simulink model "FLController_a_diff"  (R2018a)
settings: Solver=FixedStepAuto  StartTime=0.0  StopTime=10  MaxStep=0.01  RelTol=1e-4  EnableMultiTasking=on
libraries: fuzblock x4
settings Model: Creator=G  LastModifiedBy=G
settings DataIOCC: LimitDataPoints=on  SaveOutput=off  SaveTime=off
settings OptimizationCC: ExpressionDepthLimit=2147483647  LifeSpan=1
settings DebuggingCC: UnderspecifiedInitializationDetection=Classic  MergeDetectMultiDrivingBlocksExec=none  FcnCallInpInsideContextMsg=warning  AllowSymbolicDim=off  StateNameClashWarn=warning  SFUnexpectedBacktrackingDiag=warning  SFNoUnconditionalDefaultTransitionDiag=warning  SFExecutionAtInitializationDiag=none
settings CodeAppCC: StateflowObjectComments=on
settings GRTTargetCC: TargetLangStandard=C89/C90 (ANSI)  GeneratePreprocessorConditionals=Disable all  CombineOutputUpdateFcns=off  GRTInterface=on

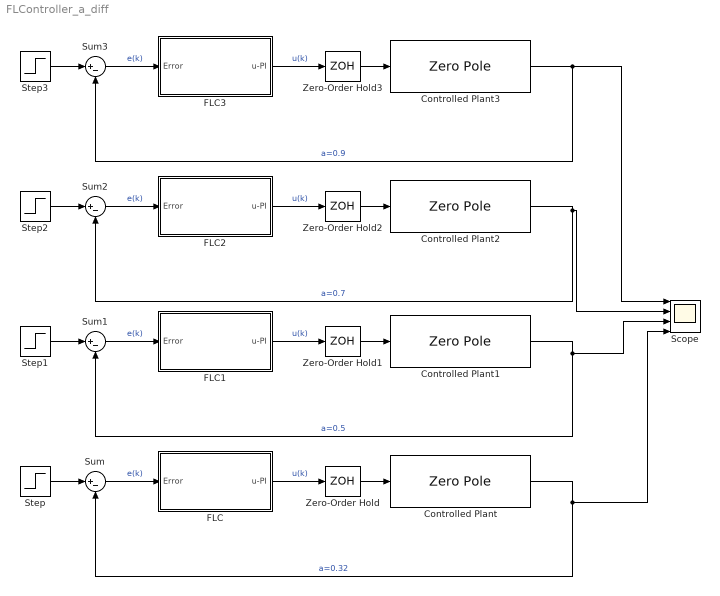
== system FLController_a_diff ==
  Controlled Plant{,1..3} (4 alike) : ZeroPole  Zeros=[]  Poles=[-0.1 -10]  Gain=25
  FLC : Subsystem
  FLC1 : Subsystem
  FLC2 : Subsystem
  FLC3 : Subsystem
  Scope : Scope  NumInputPorts=4
  Step{,1..3} (4 alike) : Step  Time=0  After=50  SampleTime=0.01
  Sum{,1..3} (4 alike) : Sum  Inputs=|+-
  Zero-Order Hold{,1..3} (4 alike) : ZeroOrderHold  SampleTime=-1
  wires:
  Controlled Plant/1 -> Scope/4, Sum/2  "a=0.32"
  Sum/1 -> FLC/1(Error)  "e(k)"
  FLC/1(u-PI) -> Zero-Order Hold/1  "u(k)"
  Zero-Order Hold/1 -> Controlled Plant/1
  Step/1 -> Sum/1
  Step1/1 -> Sum1/1
  Zero-Order Hold1/1 -> Controlled Plant1/1
  FLC1/1(u-PI) -> Zero-Order Hold1/1  "u(k)"
  Sum1/1 -> FLC1/1(Error)  "e(k)"
  Controlled Plant1/1 -> Scope/3, Sum1/2  "a=0.5"
  Step2/1 -> Sum2/1
  Zero-Order Hold2/1 -> Controlled Plant2/1
  FLC2/1(u-PI) -> Zero-Order Hold2/1  "u(k)"
  Sum2/1 -> FLC2/1(Error)  "e(k)"
  Controlled Plant2/1 -> Scope/2, Sum2/2  "a=0.7"
  Step3/1 -> Sum3/1
  Zero-Order Hold3/1 -> Controlled Plant3/1
  FLC3/1(u-PI) -> Zero-Order Hold3/1  "u(k)"
  Sum3/1 -> FLC3/1(Error)  "e(k)"
  Controlled Plant3/1 -> Scope/1, Sum3/2  "a=0.9"

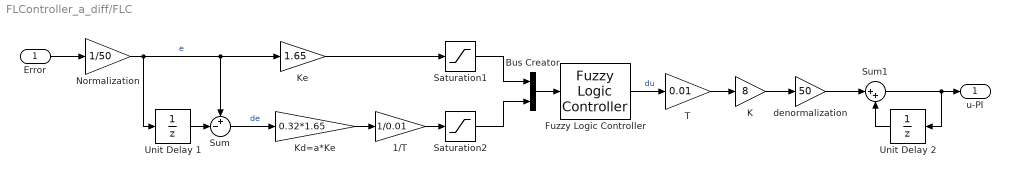
== system FLController_a_diff/FLC ==
  Error : Inport
  "1/T " : Gain  Gain=1/0.01
  Bus Creator : BusCreator  Inputs=2
  Fuzzy Logic Controller : fuzblock/Fuzzy Logic  Controller  FIS='FLController.fis'  OutputSampleNumber=101  DataType=double  FuzzifiedInputs=off  RuleFiringStrengths=off  RuleOutputs=off  AggregatedOutputs=off  SimulateUsing=Interpreted execution  OutOfRangeInputValueMessage=warning  NoRuleFiredMessage=warning  EmptyOutputFuzzySetMessage=warning
  K : Gain  Gain=8
  Kd=a*Ke : Gain  Gain=0.32*1.65
  Ke : Gain  Gain=1.65
  Normalization : Gain  Gain=1/50
  Saturation1 : Saturate  UpperLimit=1  LowerLimit=-1
  Saturation2 : Saturate  UpperLimit=1  LowerLimit=-1
  Sum : Sum  Inputs=+-|
  Sum1 : Sum  Inputs=|++
  T : Gain  Gain=0.01
  Unit Delay 1 : UnitDelay  SampleTime=-1
  Unit Delay 2 : UnitDelay  SampleTime=-1
  denormalization : Gain  Gain=50
  u-PI : Outport
  wires:
  Error/1 -> Normalization/1
  Normalization/1 -> Sum/1, Ke/1, Unit Delay 1/1  "e"
  Unit Delay 1/1 -> Sum/2
  Sum/1 -> Kd=a*Ke/1  "de"
  Kd=a*Ke/1 -> "1/T "/1
  "1/T "/1 -> Saturation2/1
  Ke/1 -> Saturation1/1
  Saturation1/1 -> Bus Creator/1
  Saturation2/1 -> Bus Creator/2
  Bus Creator/1 -> Fuzzy Logic Controller/1
  Fuzzy Logic Controller/1 -> T/1  "du"
  T/1 -> K/1
  K/1 -> denormalization/1
  denormalization/1 -> Sum1/1
  Unit Delay 2/1 -> Sum1/2
  Sum1/1 -> Unit Delay 2/1, u-PI/1

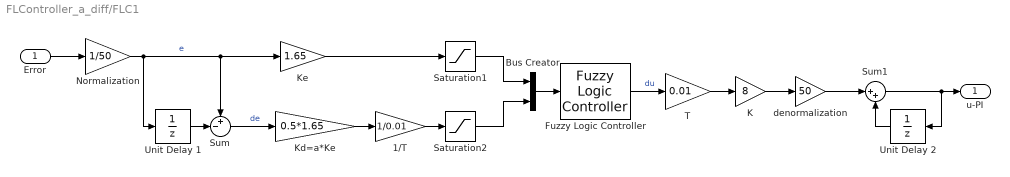
== system FLController_a_diff/FLC1 ==
  Error : Inport
  "1/T " : Gain  Gain=1/0.01
  Bus Creator : BusCreator  Inputs=2
  Fuzzy Logic Controller : fuzblock/Fuzzy Logic  Controller  FIS='FLController.fis'  OutputSampleNumber=101  DataType=double  FuzzifiedInputs=off  RuleFiringStrengths=off  RuleOutputs=off  AggregatedOutputs=off  SimulateUsing=Interpreted execution  OutOfRangeInputValueMessage=warning  NoRuleFiredMessage=warning  EmptyOutputFuzzySetMessage=warning
  K : Gain  Gain=8
  Kd=a*Ke : Gain  Gain=0.5*1.65
  Ke : Gain  Gain=1.65
  Normalization : Gain  Gain=1/50
  Saturation1 : Saturate  UpperLimit=1  LowerLimit=-1
  Saturation2 : Saturate  UpperLimit=1  LowerLimit=-1
  Sum : Sum  Inputs=+-|
  Sum1 : Sum  Inputs=|++
  T : Gain  Gain=0.01
  Unit Delay 1 : UnitDelay  SampleTime=-1
  Unit Delay 2 : UnitDelay  SampleTime=-1
  denormalization : Gain  Gain=50
  u-PI : Outport
  wires:
  Error/1 -> Normalization/1
  Normalization/1 -> Sum/1, Ke/1, Unit Delay 1/1  "e"
  Unit Delay 1/1 -> Sum/2
  Sum/1 -> Kd=a*Ke/1  "de"
  Kd=a*Ke/1 -> "1/T "/1
  "1/T "/1 -> Saturation2/1
  Ke/1 -> Saturation1/1
  Saturation1/1 -> Bus Creator/1
  Saturation2/1 -> Bus Creator/2
  Bus Creator/1 -> Fuzzy Logic Controller/1
  Fuzzy Logic Controller/1 -> T/1  "du"
  T/1 -> K/1
  K/1 -> denormalization/1
  denormalization/1 -> Sum1/1
  Unit Delay 2/1 -> Sum1/2
  Sum1/1 -> Unit Delay 2/1, u-PI/1

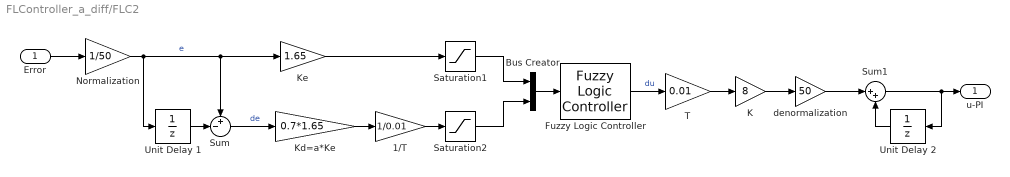
== system FLController_a_diff/FLC2 ==
  Error : Inport
  "1/T " : Gain  Gain=1/0.01
  Bus Creator : BusCreator  Inputs=2
  Fuzzy Logic Controller : fuzblock/Fuzzy Logic  Controller  FIS='FLController.fis'  OutputSampleNumber=101  DataType=double  FuzzifiedInputs=off  RuleFiringStrengths=off  RuleOutputs=off  AggregatedOutputs=off  SimulateUsing=Interpreted execution  OutOfRangeInputValueMessage=warning  NoRuleFiredMessage=warning  EmptyOutputFuzzySetMessage=warning
  K : Gain  Gain=8
  Kd=a*Ke : Gain  Gain=0.7*1.65
  Ke : Gain  Gain=1.65
  Normalization : Gain  Gain=1/50
  Saturation1 : Saturate  UpperLimit=1  LowerLimit=-1
  Saturation2 : Saturate  UpperLimit=1  LowerLimit=-1
  Sum : Sum  Inputs=+-|
  Sum1 : Sum  Inputs=|++
  T : Gain  Gain=0.01
  Unit Delay 1 : UnitDelay  SampleTime=-1
  Unit Delay 2 : UnitDelay  SampleTime=-1
  denormalization : Gain  Gain=50
  u-PI : Outport
  wires:
  Error/1 -> Normalization/1
  Normalization/1 -> Sum/1, Ke/1, Unit Delay 1/1  "e"
  Unit Delay 1/1 -> Sum/2
  Sum/1 -> Kd=a*Ke/1  "de"
  Kd=a*Ke/1 -> "1/T "/1
  "1/T "/1 -> Saturation2/1
  Ke/1 -> Saturation1/1
  Saturation1/1 -> Bus Creator/1
  Saturation2/1 -> Bus Creator/2
  Bus Creator/1 -> Fuzzy Logic Controller/1
  Fuzzy Logic Controller/1 -> T/1  "du"
  T/1 -> K/1
  K/1 -> denormalization/1
  denormalization/1 -> Sum1/1
  Unit Delay 2/1 -> Sum1/2
  Sum1/1 -> Unit Delay 2/1, u-PI/1

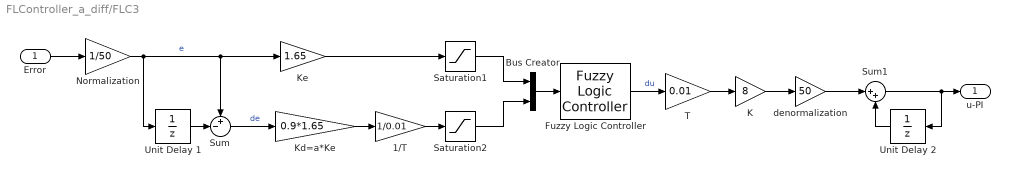
== system FLController_a_diff/FLC3 ==
  Error : Inport
  "1/T " : Gain  Gain=1/0.01
  Bus Creator : BusCreator  Inputs=2
  Fuzzy Logic Controller : fuzblock/Fuzzy Logic  Controller  FIS='FLController.fis'  OutputSampleNumber=101  DataType=double  FuzzifiedInputs=off  RuleFiringStrengths=off  RuleOutputs=off  AggregatedOutputs=off  SimulateUsing=Interpreted execution  OutOfRangeInputValueMessage=warning  NoRuleFiredMessage=warning  EmptyOutputFuzzySetMessage=warning
  K : Gain  Gain=8
  Kd=a*Ke : Gain  Gain=0.9*1.65
  Ke : Gain  Gain=1.65
  Normalization : Gain  Gain=1/50
  Saturation1 : Saturate  UpperLimit=1  LowerLimit=-1
  Saturation2 : Saturate  UpperLimit=1  LowerLimit=-1
  Sum : Sum  Inputs=+-|
  Sum1 : Sum  Inputs=|++
  T : Gain  Gain=0.01
  Unit Delay 1 : UnitDelay  SampleTime=-1
  Unit Delay 2 : UnitDelay  SampleTime=-1
  denormalization : Gain  Gain=50
  u-PI : Outport
  wires:
  Error/1 -> Normalization/1
  Normalization/1 -> Sum/1, Ke/1, Unit Delay 1/1  "e"
  Unit Delay 1/1 -> Sum/2
  Sum/1 -> Kd=a*Ke/1  "de"
  Kd=a*Ke/1 -> "1/T "/1
  "1/T "/1 -> Saturation2/1
  Ke/1 -> Saturation1/1
  Saturation1/1 -> Bus Creator/1
  Saturation2/1 -> Bus Creator/2
  Bus Creator/1 -> Fuzzy Logic Controller/1
  Fuzzy Logic Controller/1 -> T/1  "du"
  T/1 -> K/1
  K/1 -> denormalization/1
  denormalization/1 -> Sum1/1
  Unit Delay 2/1 -> Sum1/2
  Sum1/1 -> Unit Delay 2/1, u-PI/1
